simulink model "aula05_ex2"  (Simulink 7.8)
settings: Solver=ode5  StartTime=0.0  StopTime=3  RelTol=1e-3
undefined symbols (not defined in the file or in its folder): National_Instruments, PCI, pin
libraries: rtwinlib x2
settings Model: Creator=unieyiasbech  LastModifiedBy=unieyiasbech  SimulationMode=external  ExtModeTrigDuration=100000
settings HardwareCC: ProdIntDivRoundTo=Zero  ProdEndianess=LittleEndian  ProdHWDeviceType=Generic->32-bit x86 compatible
settings RTWCC: SystemTargetFile=rtwin.tlc  TemplateMakefile=rtwin.tmf  Description=Real-Time Windows Target  ProcessScript=rtwin_make_rtw_hook  RTWCompilerOptimization=On
settings CodeAppCC: MaxIdLength=95
settings RTWinTargetCC: TargetLibSuffix=_rtwin.lib  TargetPreCompLibLocation=C:\Program Files\MATLAB\R2011b\toolbox\rtw\targets\rtwin\lib\win32  TargetFunctionLibrary=ANSI_C  CodeExecutionProfiling=off  PortableWordSizes=off  RTWinDir=C:/PROGRA~1/MATLAB/R2011b/toolbox/rtw/targets/rtwin  TargetArch=win32

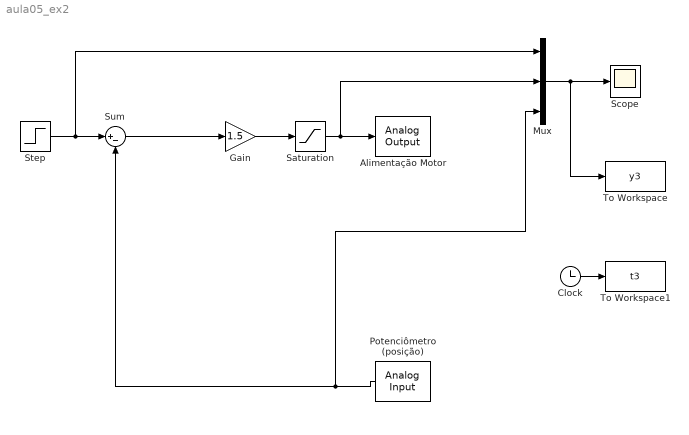
== system aula05_ex2 ==
  Alimentação Motor : rtwinlib/Analog Output  SampleTime=1/1000  DrvName=National_Instruments/PCI-6221_37-pin  DrvAddress=4294967295  DrvOptions=[0 0 0 0 0]  Channels=1  RangeMode=1  VoltRange=1  InitialValue=0  FinalValue=0
      settings: AttributesFormatString=National Instruments\nPCI-6221 37-pin [auto]
  Clock : Clock
  Gain : Gain  Gain=1.5
  Mux : Mux  Inputs=3
  Potenciômetro (posição) : rtwinlib/Analog Input  SampleTime=1/1000  DrvName=National_Instruments/PCI-6221_37-pin  DrvAddress=4294967295  DrvOptions=[0 0 0 0 0]  Channels=4  RangeMode=1  VoltRange=1  DataType=1
      settings: AttributesFormatString=National Instruments\nPCI-6221 37-pin [auto]
  Saturation : Saturate  UpperLimit=5  LowerLimit=-5
  Scope : Scope
      settings: MaxDataPoints=1010
  Step : Step  Time=2  After=2  SampleTime=0
  Sum : Sum  Inputs=|+-
  To Workspace : ToWorkspace  VariableName=y3  SampleTime=1/1000  SaveFormat=Array
  To Workspace1 : ToWorkspace  VariableName=t3  SampleTime=1/1000  SaveFormat=Array
  wires:
  Step/1 -> Sum/1, Mux/1
  Mux/1 -> Scope/1, To Workspace/1
  Saturation/1 -> Alimentação Motor/1, Mux/2
  Potenciômetro (posição)/1 -> Sum/2, Mux/3
  Gain/1 -> Saturation/1
  Clock/1 -> To Workspace1/1
  Sum/1 -> Gain/1
